simulink model "one_kanal"  (R2024a)
settings: Solver=VariableStepAuto  StartTime=0.0  StopTime=1000  RelTol=1e-3
settings Model: Creator=evgenijkondratev  LastModifiedBy=evgenijkondratev

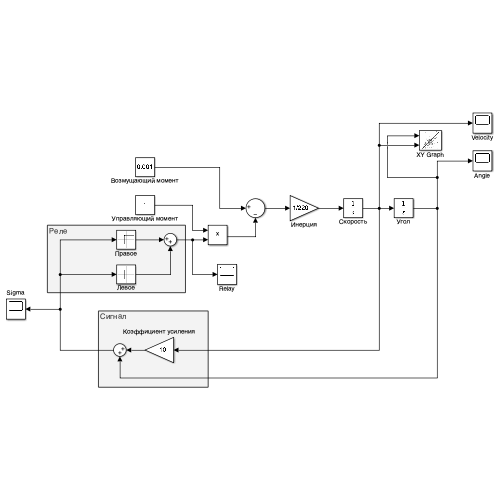
[thumbnail: Simulink's stored preview of the top-level diagram]
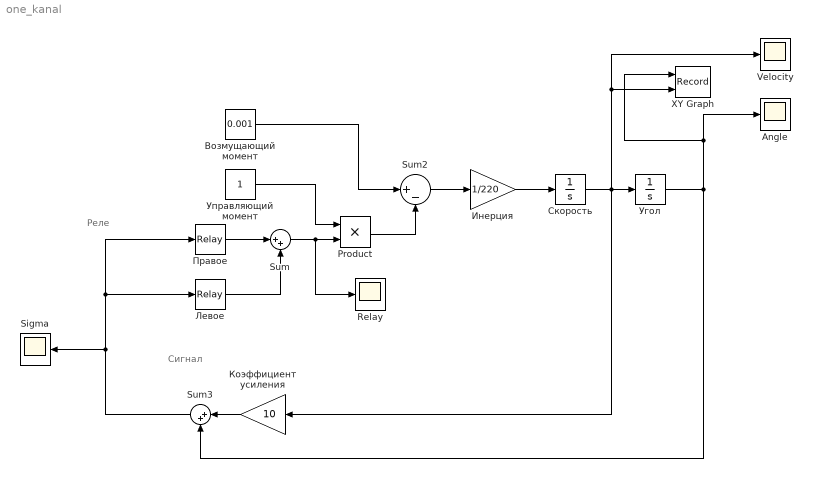
== system one_kanal ==
  note: Сигнал
  note: Реле
  Angle : Scope
  Product : Product
  Relay : Scope
  Sigma : Scope
  Sum : Sum  Inputs=|++
  Sum2 : Sum  Inputs=|+-
  Sum3 : Sum  Inputs=|++
  Velocity : Scope
  XY Graph : Record  FileSettingsInternal="{\"entries\":[{\"content\":{\"excelSettings\":{\"content\":{},\"type\":\"Streamout.ExcelSettings\"}},\"type\":\"Streamout.FileSettingStorage\",\"uuid\":\"\"}],\"packageUris\":[\"http:\\/\\/schema.mathworks.com\\/mf0\\/streamout_blocks\\/R2020a\"],\"version\":\"1.0\"}"  Layout=[1 1]  SignalsInternal="{\"entries\":[{\"content\":{\"signals\":[{\"content\":{\"blockPath\":[],\"dimensions\":[1],\"domain\":\"\",\"lineColor\":\"#a2142f\",\"plots\":[ 1 ],\"port\":1,\"sid\":[\"\"],\"signalID\":1,\"signalName\":\"Угол\"},\"type\":\"RecordBlkView.Signal\",\"uuid\":\"\"},{\"content\":{\"blockPath\":[],\"dimensions\":[1],\"domain\":\"\",\"lineColor\":\"#139fff\",\"plots\":[ 1 ],\"port\":2,\"sid\":[\"\"],\"signalID\":2,\"signalName\":\"Скорость\"},\"type\":\"RecordBlkView.Signal\",\"uuid\":\"\"}]},\"type\":\"RecordBlkView.InputSignals\",\"uuid\":\"\"}],\"packageUris\":[\"http:\\/\\/schema.mathworks.com\\/mf0\\/streamout_blocks\\/R2020a\"],\"version\":\"1.0\"}"  VisualizationBindings="{\"xyplotplugin\":{\"info\":[{\"series\":[{\"bindingParametersList\":[{\"parameter\":\"X-Axis\",\"signalID\":1,\"signalName\":\"Угол\"},{\"parameter\":\"Y-Axis\",\"signalID\":2,\"signalName\":\"Скорость\"},{\"parameter\":\"X-Axis\",\"signalID\":1,\"signalName\":\"Угол\"},{\"parameter\":\"Y-Axis\",\"signalID\":2,\"signalName\":\"Скорость\"},{\"parameter\":\"X-Axis\",\"signalID\":1,\"signalName\":\"Угол\"},{\"parameter\":\"Y-Axis\",\"signalID\":2,\"signalName\":\"Скорость\"},{\"parameter\":\"X-Axis\",\"signalID\":1,\"signalName\":\"Угол\"},{\"parameter\":\"Y-Axis\",\"signalID\":2,\"signalName\":\"Скорость\"},{\"parameter\":\"X-Axis\",\"signalID\":1,\"signalName\":\"Угол\"},{\"parameter\":\"Y-Axis\",\"signalID\":2,\"signalName\":\"Скорость\"}],\"seriesID\":0}],\"subplotID\":1}]}}"  CompatibilityTag=XY
  Возмущающий момент : Constant  Value=0.001
  Инерция : Gain  Gain=1/220
  Коэффициент усиления : Gain  Gain=10
  Левое : Relay  OnSwitchValue=-0.08  OffSwitchValue=-1  OnOutputValue=0  OffOutputValue=-1
  Правое : Relay  OnSwitchValue=0.1  OffSwitchValue=0.08
  Скорость : Integrator  InitialCondition=0.001
  Угол : Integrator  InitialCondition=0.001
  Управляющий момент : Constant
  wires:
  Правое/1 -> Sum/1
  Левое/1 -> Sum/2
  Sum/1 -> Relay/1, Product/2
  Sum3/1 -> Левое/1, Правое/1, Sigma/1
  Управляющий момент/1 -> Product/1
  Product/1 -> Sum2/2
  Возмущающий момент/1 -> Sum2/1
  Sum2/1 -> Инерция/1
  Инерция/1 -> Скорость/1
  Скорость/1 -> XY Graph/2, Velocity/1, Угол/1, Коэффициент усиления/1
  Коэффициент усиления/1 -> Sum3/1
  Угол/1 -> XY Graph/1, Angle/1, Sum3/2
